simulink model "bai2"  (R2017b)
settings: Solver=ode5  StartTime=0.0  StopTime=60  FixedStep=0.01  RelTol=1e-3
libraries: fuzblock x1
settings Model: Creator=phamt  LastModifiedBy=phamt

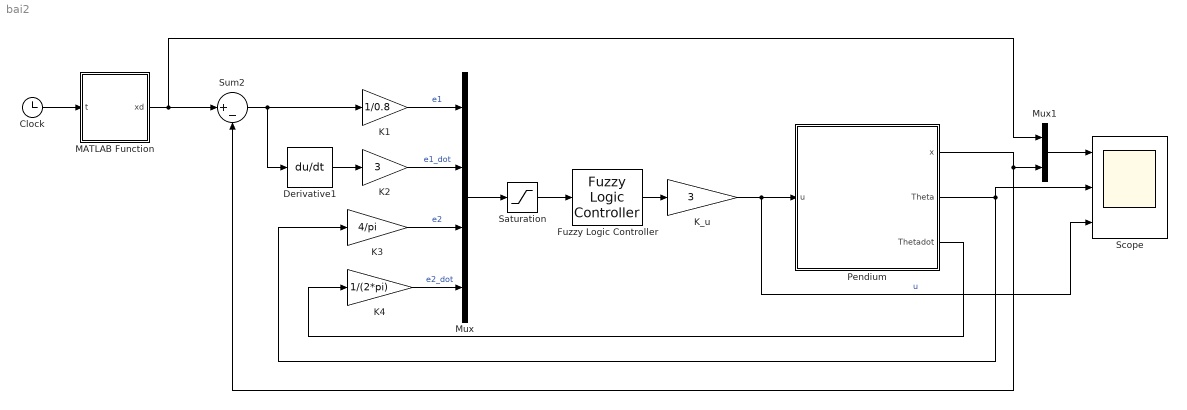
== system bai2 ==
  Clock : Clock
      settings: Decimation=60
  Derivative1 : Derivative
  Fuzzy Logic Controller : fuzblock/Fuzzy Logic  Controller  FIS='bai2_FIS.fis'  OutputSampleNumber=101  DataType=double  FuzzifiedInputs=off  RuleFiringStrengths=off  RuleOutputs=off  AggregatedOutputs=off  SimulateUsing=Interpreted execution
  K1 : Gain  Gain=1/0.8
  K2 : Gain  Gain=3
  K3 : Gain  Gain=4/pi
  K4 : Gain  Gain=1/(2*pi)
  K_u : Gain  Gain=3
  MATLAB Function : MATLAB Function  TreatAsAtomicUnit=on
  Mux : Mux
  Mux1 : Mux  Inputs=2
  Pendium : Subsystem  mask{H=0.5, m=2, l=0.6, g=9.81, x0=0.2, xdot0=0.001, theta0=pi/36, thetadot0=pi/18}
      mask prompts: H "M"
  Saturation : Saturate  UpperLimit=1  LowerLimit=-1
  Scope : Scope  NumInputPorts=3
  Sum2 : Sum  Inputs=|+-
  wires:
  Sum2/1 -> Derivative1/1, K1/1
  Saturation/1 -> Fuzzy Logic Controller/1
  Mux/1 -> Saturation/1
  Derivative1/1 -> K2/1
  Fuzzy Logic Controller/1 -> K_u/1
  K3/1 -> Mux/3  "e2"
  K2/1 -> Mux/2  "e1_dot"
  Clock/1 -> MATLAB Function/1(t)
  K1/1 -> Mux/1  "e1"
  K4/1 -> Mux/4  "e2_dot"
  K_u/1 -> Scope/3, Pendium/1(u)  "u"
  Pendium/3(Thetadot) -> K4/1
  Pendium/2(Theta) -> Scope/2, K3/1
  MATLAB Function/1(xd) -> Mux1/1, Sum2/1
  Mux1/1 -> Scope/1
  Pendium/1(x) -> Mux1/2, Sum2/2

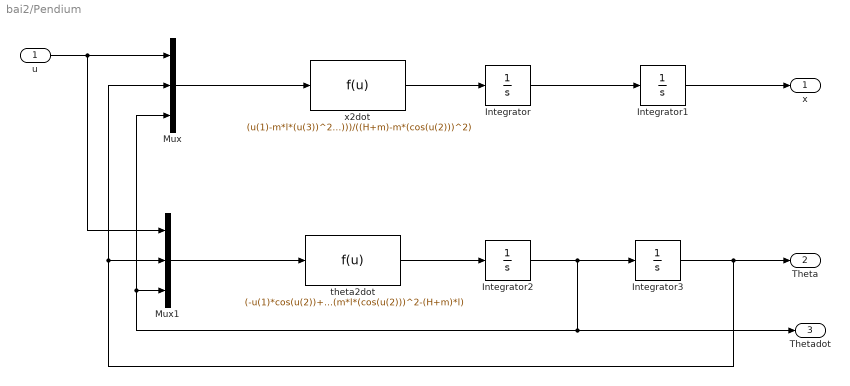
== system bai2/Pendium ==
  u : Inport
  Integrator : Integrator  InitialCondition=xdot0
  Integrator1 : Integrator  InitialCondition=x0
  Integrator2 : Integrator  InitialCondition=thetadot0
  Integrator3 : Integrator  InitialCondition=theta0
  Mux : Mux  Inputs=3
  Mux1 : Mux  Inputs=3
  theta2dot : Fcn  Expr=(-u(1)*cos(u(2))+m*g*(u(3))^2*sin(u(2))*cos(u(2))+(H+m)*(g*sin(u(2))))/(m*l*(cos(u(2)))^2-(H+m)*l)
  x2dot : Fcn  Expr=(u(1)-m*l*(u(3))^2*sin(u(2))-m*g*sin(u(2))*cos(u(2)))/((H+m)-m*(cos(u(2)))^2)
  x : Outport
  Theta : Outport  Port=2
  Thetadot : Outport  Port=3
  wires:
  u/1 -> Mux1/1, Mux/1
  Mux/1 -> x2dot/1
  x2dot/1 -> Integrator/1
  Integrator/1 -> Integrator1/1
  Mux1/1 -> theta2dot/1
  Integrator2/1 -> Mux/3, Mux1/3, Thetadot/1, Integrator3/1
  theta2dot/1 -> Integrator2/1
  Integrator1/1 -> x/1
  Integrator3/1 -> Mux/2, Mux1/2, Theta/1

== matlab function bai2/MATLAB Function ==
  data: t input; xd output
function xd = fcn(t)
if (0<=t) && (t<10)  
    xd = 0.45;
elseif (10<=t) &&(t<20) 
    xd = 0.2;
elseif (20<=t) &&(t<30)  
    xd = 0.8;
elseif (30<=t) &&(t<40)  
    xd = 0.55;
elseif (40<=t) &&(t<50)  
    xd = 0.1;
elseif (50<=t) &&(t<60)  
    xd = 0.65;
else xd = 0;
end
end
